simulink model "modelsimulator"  (R2023b)
settings: Solver=VariableStepAuto  StartTime=0.0  StopTime=185  FixedStep=0.0002  RelTol=1e-3
values from neighbouring files (symbols this model uses):
  eta_init = [0 0 0 0 0 0]    [Linearization_validation.m]    (also in ROV_simulation_init.m = [radius 0 0 0 0 -pi/2])
  K_full = lqr(linsysROV_lqr,Q,R)    [ROV_simulation_init.m]
  K_reduced = lqr(linsysROV_lqr_reduced_disc,Q,R)    [ROV_simulation_init.m]
  omega = 0.0174532925*5    (= 0.0872664625)    [ROV_simulation_init.m]
  p = [-125.691529893755	-8.50647884753240	275.922008410927	13.4112646958028	-226.567986780204	-3.28875901062827	118.657519470084	6.62648580653865	14.9826070833980	0.00]    [ROV_simulation_init.m]
  PID_phi = [11.6676, 5.8503, -12.3688, 0.025226,34]    [ROV_simulation_init.m]
  PID_psi = [11.3054, 1.000, -3.8005, 0.087502,30]    [ROV_simulation_init.m]
  PID_theta = [10.2974, 5.9702, -15.653, 0.016423,19]    [ROV_simulation_init.m]
  PID_x = [500.411, 30.5093, -500.8638, 0.032394,110]    [ROV_simulation_init.m]
  PID_y = [500.7275, 20.1075, -500.8002, 0.019369,110]    [ROV_simulation_init.m]
  PID_z = [500.7655, 25.0859, -500.5557, 0.026709,158]    [ROV_simulation_init.m]
  radius = 5    [ROV_simulation_init.m]
  ROV = initializeModelMatrices(m,I,COG,l,w,h,Thrusters)    [CreateGramianROV.m]    (also in CreateROVLin.m = initializeModelMatrices(m, I, COB, dim, BlueROVHeavy); Eigenvalue_tracking.m = initializeModelMatrices(m, I, COB,dim,0); Linearization_validation.m = initializeModelMatrices(m, I, COB,dim,0); ROV_simulation_init.m = initializeModelMatrices(m, Inertia, COB, dim, BlueROVHeavy))
  T_inv = ROV.T'/(ROV.T*ROV.T')    [ROV_simulation_init.m]
  ThrusterVoltage = 14    [ROV_simulation_init.m]
  v_init = [3 0 0 0 0 0]    [Linearization_validation.m]    (also in ROV_simulation_init.m = [omega omega z_rate 0 0 omega])
  z_rate = 0.1    [ROV_simulation_init.m]
libraries: simulink x60
(part 1 of 3)
settings Model: Creator=Tomas  LastModifiedBy=Ottol

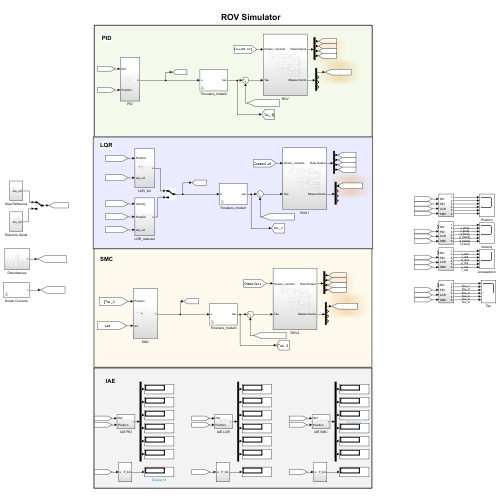
[thumbnail: Simulink's stored preview of the top-level diagram]
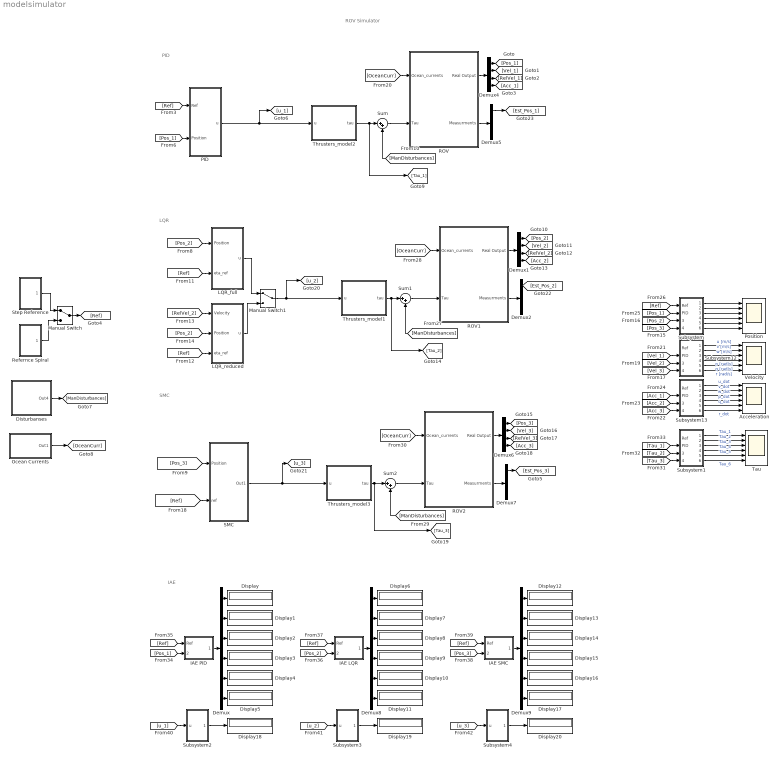
== system modelsimulator ==
  note: PID
  note: LQR
  note: SMC
  note: IAE
  note: ROV Simulator
  Acceleration : Scope  NumInputPorts=6
  Demux : Demux  Outputs=6
  Demux{1..2,4..7} (6 alike) : Demux
  Demux8 : Demux  Outputs=6
  Demux9 : Demux  Outputs=6
  Display{,1..20} (21 alike) : Display
  Disturbanses : Subsystem
  IAE LQR : Subsystem
  IAE PID : Subsystem
  IAE SMC : Subsystem
  LQR_full : Subsystem
  LQR_reduced : Subsystem
  Manual Switch : ManualSwitch
  Manual Switch1 : ManualSwitch
  Ocean Currents : Subsystem  mask{N=0, E=0, D=0}
      mask prompts: N "Current North"; E "Current East"; D "Current Down"
  PID : Subsystem
  Position : Scope  NumInputPorts=6
  ROV : Subsystem
  ROV1 : Subsystem
  ROV2 : Subsystem
  Refernce Spiral : Subsystem
  SMC : Subsystem
  Step Reference : Subsystem
  Subsystem : Subsystem
  Subsystem1 : Subsystem
  Subsystem12 : Subsystem
  Subsystem13 : Subsystem
  Subsystem2 : Subsystem
  Subsystem3 : Subsystem
  Subsystem4 : Subsystem
  Sum : Sum  Inputs=|++
  Sum1 : Sum  Inputs=|++
  Sum2 : Sum  Inputs=|++
  Tau : Scope  NumInputPorts=6
  Thrusters_model1 : Subsystem  mask{Thruster_voltage=14 V, Enable_dynamics=on}
      mask prompts: Enable_dynamics "Enable Thruster Dynamics"
      mask DialogControl DescGroupVar Prompt: T200 Thruster
      mask DialogControl DescTextVar Prompt: Thruster dynamics available for 10 to 20 V
      mask DialogControl Container3 Prompt: Thruster Voltage selection
  Thrusters_model2 : Subsystem  mask{Thruster_voltage=14 V, Enable_dynamics=on}
      mask prompts: Enable_dynamics "Enable Thruster Dynamics"
      mask DialogControl DescGroupVar Prompt: T200 Thruster
      mask DialogControl DescTextVar Prompt: Thruster dynamics available for 10 to 20 V
      mask DialogControl Container3 Prompt: Thruster Voltage selection
  Thrusters_model3 : Subsystem  mask{Thruster_voltage=14 V, Enable_dynamics=on}
      mask prompts: Enable_dynamics "Enable Thruster Dynamics"
      mask DialogControl DescGroupVar Prompt: T200 Thruster
      mask DialogControl DescTextVar Prompt: Thruster dynamics available for 10 to 20 V
      mask DialogControl Container3 Prompt: Thruster Voltage selection
  Velocity : Scope  NumInputPorts=6
  wires:
  Subsystem12/6(Out6) -> Velocity/6  "r [rad/s]"
  Subsystem12/5(Out5) -> Velocity/5  "q [rad/s]"
  Subsystem12/4(Out4) -> Velocity/4  "p [rad/s]"
  Subsystem12/3(Out3) -> Velocity/3  "w [m/s]"
  Subsystem12/2(Out2) -> Velocity/2  "v [m/s]"
  Subsystem12/1(Out1) -> Velocity/1  "u [m/s]"
  Subsystem13/1(Out1) -> Acceleration/1  "u_dot"
  Subsystem13/2(Out2) -> Acceleration/2  "v_dot"
  Subsystem13/3(Out3) -> Acceleration/3  "w_dot"
  Subsystem13/4(Out4) -> Acceleration/4  "p_dot"
  Subsystem13/5(Out5) -> Acceleration/5  "q_dot"
  Subsystem13/6(Out6) -> Acceleration/6  "r_dot"
  Sum/1 -> ROV/2(Tau)
  Thrusters_model2/1(tau) -> Sum/1, [Tau_1]
  ROV/2(Measurments) -> Demux5/1
  Subsystem/1(Out1) -> Position/1
  Subsystem/6(Out6) -> Position/6
  Subsystem/5(Out5) -> Position/5
  Subsystem/4(Out4) -> Position/4
  Subsystem/3(Out3) -> Position/3
  Subsystem/2(Out2) -> Position/2
  [Pos_1] -> PID/2(Position)
  Refernce Spiral/1(eta_ref) -> Manual Switch/2
  [Ref] -> LQR_full/2(eta_ref)
  [Ref] -> SMC/2(ref)
  Ocean Currents/1(Out1) -> [OceanCurr]
  [OceanCurr] -> ROV/1(Ocean_currents)
  Demux4/1 -> [Pos_1]
  Demux4/3 -> [RelVel_1]
  Demux4/2 -> [Vel_1]
  Demux4/4 -> [Acc_1]
  ROV/1(Real Output) -> Demux4/1
  Disturbanses/1(Out4) -> [ManDisturbances]
  [ManDisturbances] -> Sum/2
  [Pos_1] -> Subsystem/2(PID)
  [Ref] -> Subsystem/1(Ref)
  [ManDisturbances] -> Sum1/2
  ROV1/1(Real Output) -> Demux1/1
  Demux1/4 -> [Acc_2]
  Demux1/2 -> [Vel_2]
  Demux1/3 -> [RelVel_2]
  Demux1/1 -> [Pos_2]
  [OceanCurr] -> ROV1/1(Ocean_currents)
  ROV1/2(Measurments) -> Demux2/1
  Thrusters_model1/1(tau) -> [Tau_2], Sum1/1
  Sum1/1 -> ROV1/2(Tau)
  Sum2/1 -> ROV2/2(Tau)
  Thrusters_model3/1(tau) -> [Tau_3], Sum2/1
  ROV2/2(Measurments) -> Demux7/1
  [OceanCurr] -> ROV2/1(Ocean_currents)
  Demux6/1 -> [Pos_3]
  Demux6/3 -> [RelVel_3]
  Demux6/2 -> [Vel_3]
  Demux6/4 -> [Acc_3]
  ROV2/1(Real Output) -> Demux6/1
  [ManDisturbances] -> Sum2/2
  Step Reference/1(eta_ref) -> Manual Switch/1
  Manual Switch/1 -> [Ref]
  [Ref] -> PID/1(Ref)
  [Pos_2] -> LQR_full/1(Position)
  [Pos_3] -> SMC/1(Position)
  [Pos_2] -> LQR_reduced/2(Position)
  [RelVel_2] -> LQR_reduced/1(Velocity)
  [Ref] -> LQR_reduced/3(eta_ref)
  LQR_full/1(u) -> Manual Switch1/1
  LQR_reduced/1(u) -> Manual Switch1/2
  [Pos_3] -> Subsystem/4(SMC)
  [Vel_1] -> Subsystem12/2(PID)
  [Vel_2] -> Subsystem12/3(LQR)
  [Vel_3] -> Subsystem12/4(SMC)
  [Acc_1] -> Subsystem13/2(PID)
  [Acc_2] -> Subsystem13/3(LQR)
  [Acc_3] -> Subsystem13/4(SMC)
  [Tau_2] -> Subsystem1/3(LQR)
  Subsystem1/5(Out5) -> Tau/5  "Tau_5"
  Subsystem1/6(Out6) -> Tau/6  "Tau_6"
  Subsystem1/4(Out4) -> Tau/4  "Tau_4"
  Subsystem1/3(Out3) -> Tau/3  "Tau_3"
  [Tau_1] -> Subsystem1/2(PID)
  Subsystem1/1(Out1) -> Tau/1  "Tau_1"
  [Tau_3] -> Subsystem1/4(SMC)
  Subsystem1/2(Out2) -> Tau/2  "Tau_2"
  Demux/3 -> Display2/1
  Demux/1 -> Display/1
  Demux/6 -> Display5/1
  Demux/4 -> Display3/1
  Demux/2 -> Display1/1
  Demux/5 -> Display4/1
  IAE PID/1(Out1) -> Demux/1
  [Ref] -> IAE PID/1(Ref)
  [Pos_1] -> IAE PID/2(Position)
  Demux8/5 -> Display10/1
  Demux8/2 -> Display7/1
  Demux8/3 -> Display8/1
  Demux8/1 -> Display6/1
  IAE LQR/1(Out1) -> Demux8/1
  Demux8/6 -> Display11/1
  [Pos_2] -> IAE LQR/2(Position)
  Demux8/4 -> Display9/1
  [Ref] -> IAE LQR/1(Ref)
  Demux9/5 -> Display16/1
  Demux9/2 -> Display13/1
  Demux9/3 -> Display14/1
  Demux9/1 -> Display12/1
  IAE SMC/1(Out1) -> Demux9/1
  Demux9/6 -> Display17/1
  [Pos_3] -> IAE SMC/2(Position)
  Demux9/4 -> Display15/1
  [Ref] -> IAE SMC/1(Ref)
  [Pos_2] -> Subsystem/3(LQR)
  SMC/1(Out1) -> [u_3], Thrusters_model3/1(u)
  Manual Switch1/1 -> [u_2], Thrusters_model1/1(u)
  PID/1(u) -> Thrusters_model2/1(u), [u_1]
  [u_1] -> Subsystem2/1(u)
  Subsystem2/1(F_tot) -> Display18/1
  [u_2] -> Subsystem3/1(u)
  Subsystem3/1(F_tot) -> Display19/1
  [u_3] -> Subsystem4/1(u)
  Subsystem4/1(F_tot) -> Display20/1
  Demux7/1 -> [Est_Pos_3]
  Demux2/1 -> [Est_Pos_2]
  Demux5/1 -> [Est_Pos_1]

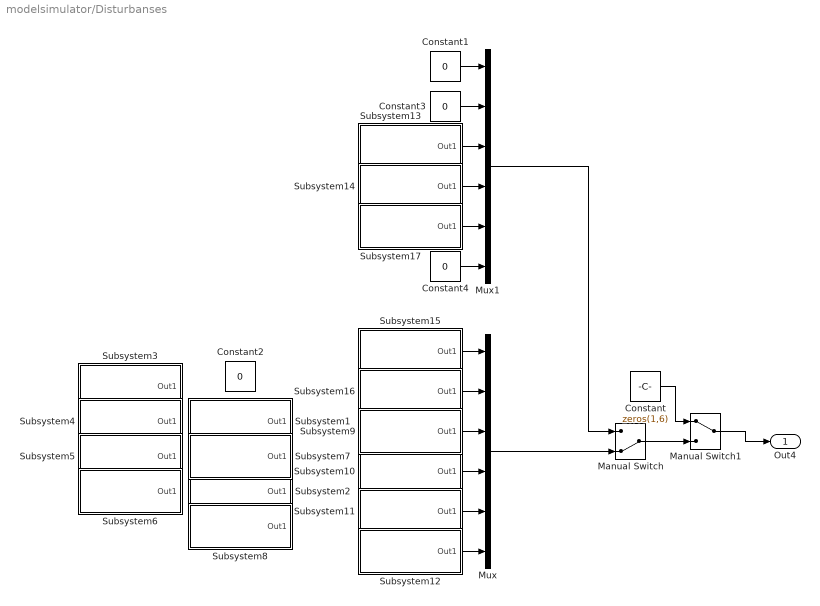
== system modelsimulator/Disturbanses ==
  Constant : Constant  Value=zeros(1,6)
  Constant{1..4} (4 alike) : Constant  Value=0
  Manual Switch : ManualSwitch  CurrentSetting=0
  Manual Switch1 : ManualSwitch
  Mux : Mux  Inputs=6
  Mux1 : Mux  Inputs=6
  Subsystem1 : Subsystem  mask{Step_time_1=5, Step_time_2=20, Init_val=0, New_val=100}
      mask prompts: Step_time_1 "Step time 1:"; Step_time_2 "Step time 2:"; Init_val "Inital Value:"; New_val "New Value:"
      mask Display: plot([1 2 3 4 4 5 6 7 7 8 9 10],[0 0 0 0 1 1 1 1 0 0 0 0]);
  Subsystem10 : Subsystem  mask{Step_time_1=95, Step_time_2=110, Init_val=0, New_val=1}
      mask prompts: Step_time_1 "Step time 1:"; Step_time_2 "Step time 2:"; Init_val "Inital Value:"; New_val "New Value:"
      mask Display: plot([1 2 3 4 4 5 6 7 7 8 9 10],[0 0 0 0 1 1 1 1 0 0 0 0]);
  Subsystem11 : Subsystem  mask{Step_time_1=125, Step_time_2=140, Init_val=0, New_val=1}
      mask prompts: Step_time_1 "Step time 1:"; Step_time_2 "Step time 2:"; Init_val "Inital Value:"; New_val "New Value:"
      mask Display: plot([1 2 3 4 4 5 6 7 7 8 9 10],[0 0 0 0 1 1 1 1 0 0 0 0]);
  Subsystem12 : Subsystem  mask{Step_time_1=155, Step_time_2=170, Init_val=0, New_val=1}
      mask prompts: Step_time_1 "Step time 1:"; Step_time_2 "Step time 2:"; Init_val "Inital Value:"; New_val "New Value:"
      mask Display: plot([1 2 3 4 4 5 6 7 7 8 9 10],[0 0 0 0 1 1 1 1 0 0 0 0]);
  Subsystem13 : Subsystem  mask{Step_time_1=95, Step_time_2=110, Init_val=0, New_val=10}
      mask prompts: Step_time_1 "Step time 1:"; Step_time_2 "Step time 2:"; Init_val "Inital Value:"; New_val "New Value:"
      mask Display: plot([1 2 3 4 4 5 6 7 7 8 9 10],[0 0 0 0 1 1 1 1 0 0 0 0]);
  Subsystem14 : Subsystem  mask{Step_time_1=125, Step_time_2=140, Init_val=0, New_val=1}
      mask prompts: Step_time_1 "Step time 1:"; Step_time_2 "Step time 2:"; Init_val "Inital Value:"; New_val "New Value:"
      mask Display: plot([1 2 3 4 4 5 6 7 7 8 9 10],[0 0 0 0 1 1 1 1 0 0 0 0]);
  Subsystem15 : Subsystem  mask{Step_time_1=5, Step_time_2=20, Init_val=0, New_val=10}
      mask prompts: Step_time_1 "Step time 1:"; Step_time_2 "Step time 2:"; Init_val "Inital Value:"; New_val "New Value:"
      mask Display: plot([1 2 3 4 4 5 6 7 7 8 9 10],[0 0 0 0 1 1 1 1 0 0 0 0]);
  Subsystem16 : Subsystem  mask{Step_time_1=35, Step_time_2=50, Init_val=0, New_val=10}
      mask prompts: Step_time_1 "Step time 1:"; Step_time_2 "Step time 2:"; Init_val "Inital Value:"; New_val "New Value:"
      mask Display: plot([1 2 3 4 4 5 6 7 7 8 9 10],[0 0 0 0 1 1 1 1 0 0 0 0]);
  Subsystem17 : Subsystem  mask{Step_time_1=155, Step_time_2=170, Init_val=0, New_val=1}
      mask prompts: Step_time_1 "Step time 1:"; Step_time_2 "Step time 2:"; Init_val "Inital Value:"; New_val "New Value:"
      mask Display: plot([1 2 3 4 4 5 6 7 7 8 9 10],[0 0 0 0 1 1 1 1 0 0 0 0]);
  Subsystem2 : Subsystem  mask{Step_time_1=65, Step_time_2=80, Init_val=0, New_val=1}
      mask prompts: Step_time_1 "Step time 1:"; Step_time_2 "Step time 2:"; Init_val "Inital Value:"; New_val "New Value:"
      mask Display: plot([1 2 3 4 4 5 6 7 7 8 9 10],[0 0 0 0 1 1 1 1 0 0 0 0]);
  Subsystem3 : Subsystem  mask{Step_time_1=14, Step_time_2=16, Init_val=0, New_val=5}
      mask prompts: Step_time_1 "Step time 1:"; Step_time_2 "Step time 2:"; Init_val "Inital Value:"; New_val "New Value:"
      mask Display: plot([1 2 3 4 4 5 6 7 7 8 9 10],[0 0 0 0 1 1 1 1 0 0 0 0]);
  Subsystem4 : Subsystem  mask{Step_time_1=20, Step_time_2=22, Init_val=0, New_val=1}
      mask prompts: Step_time_1 "Step time 1:"; Step_time_2 "Step time 2:"; Init_val "Inital Value:"; New_val "New Value:"
      mask Display: plot([1 2 3 4 4 5 6 7 7 8 9 10],[0 0 0 0 1 1 1 1 0 0 0 0]);
  Subsystem5 : Subsystem  mask{Step_time_1=26, Step_time_2=28, Init_val=0, New_val=1}
      mask prompts: Step_time_1 "Step time 1:"; Step_time_2 "Step time 2:"; Init_val "Inital Value:"; New_val "New Value:"
      mask Display: plot([1 2 3 4 4 5 6 7 7 8 9 10],[0 0 0 0 1 1 1 1 0 0 0 0]);
  Subsystem6 : Subsystem  mask{Step_time_1=32, Step_time_2=34, Init_val=0, New_val=1}
      mask prompts: Step_time_1 "Step time 1:"; Step_time_2 "Step time 2:"; Init_val "Inital Value:"; New_val "New Value:"
      mask Display: plot([1 2 3 4 4 5 6 7 7 8 9 10],[0 0 0 0 1 1 1 1 0 0 0 0]);
  Subsystem7 : Subsystem  mask{Step_time_1=35, Step_time_2=50, Init_val=0, New_val=10}
      mask prompts: Step_time_1 "Step time 1:"; Step_time_2 "Step time 2:"; Init_val "Inital Value:"; New_val "New Value:"
      mask Display: plot([1 2 3 4 4 5 6 7 7 8 9 10],[0 0 0 0 1 1 1 1 0 0 0 0]);
  Subsystem8 : Subsystem  mask{Step_time_1=95, Step_time_2=110, Init_val=0, New_val=10}
      mask prompts: Step_time_1 "Step time 1:"; Step_time_2 "Step time 2:"; Init_val "Inital Value:"; New_val "New Value:"
      mask Display: plot([1 2 3 4 4 5 6 7 7 8 9 10],[0 0 0 0 1 1 1 1 0 0 0 0]);
  Subsystem9 : Subsystem  mask{Step_time_1=65, Step_time_2=80, Init_val=0, New_val=10}
      mask prompts: Step_time_1 "Step time 1:"; Step_time_2 "Step time 2:"; Init_val "Inital Value:"; New_val "New Value:"
      mask Display: plot([1 2 3 4 4 5 6 7 7 8 9 10],[0 0 0 0 1 1 1 1 0 0 0 0]);
  Out4 : Outport
  wires:
  Subsystem9/1(Out1) -> Mux/3
  Subsystem15/1(Out1) -> Mux/1
  Subsystem16/1(Out1) -> Mux/2
  Subsystem10/1(Out1) -> Mux/4
  Subsystem11/1(Out1) -> Mux/5
  Subsystem12/1(Out1) -> Mux/6
  Subsystem13/1(Out1) -> Mux1/3
  Subsystem14/1(Out1) -> Mux1/4
  Subsystem17/1(Out1) -> Mux1/5
  Constant1/1 -> Mux1/1
  Constant3/1 -> Mux1/2
  Constant4/1 -> Mux1/6
  Mux/1 -> Manual Switch/2
  Mux1/1 -> Manual Switch/1
  Manual Switch/1 -> Manual Switch1/2
  Manual Switch1/1 -> Out4/1
  Constant/1 -> Manual Switch1/1

== system modelsimulator/IAE LQR ==
  Ref : Inport
  Position : Inport  Port=2
  Abs : Abs  SaturateOnIntegerOverflow=off
  Integrator : Integrator
  Sum : Sum  Inputs=|+-
  Out1 : Outport
  wires:
  Ref/1 -> Sum/1
  Position/1 -> Sum/2
  Sum/1 -> Abs/1
  Abs/1 -> Integrator/1
  Integrator/1 -> Out1/1

== system modelsimulator/IAE PID ==
  Ref : Inport
  Position : Inport  Port=2
  Abs : Abs  SaturateOnIntegerOverflow=off
  Integrator : Integrator
  Sum : Sum  Inputs=|+-
  Out1 : Outport
  wires:
  Ref/1 -> Sum/1
  Position/1 -> Sum/2
  Sum/1 -> Abs/1
  Abs/1 -> Integrator/1
  Integrator/1 -> Out1/1

== system modelsimulator/IAE SMC ==
  Ref : Inport
  Position : Inport  Port=2
  Abs : Abs  SaturateOnIntegerOverflow=off
  Integrator : Integrator
  Sum : Sum  Inputs=|+-
  Out1 : Outport
  wires:
  Ref/1 -> Sum/1
  Position/1 -> Sum/2
  Sum/1 -> Abs/1
  Abs/1 -> Integrator/1
  Integrator/1 -> Out1/1

== system modelsimulator/LQR_full ==
  Position : Inport  PortDimensions=6
  eta_ref : Inport  Port=2  PortDimensions=6
  Constant7 : Constant  Value=-K_full
  Demux : Demux  Outputs=6
  Demux1 : Demux  Outputs=6
  Demux2 : Demux  Outputs=6
  Discrete Derivative2 : simulink/Discrete/Discrete Derivative  gainval=1.0  ICPrevScaledInput=0.0  OutMin=[]  OutMax=[]  OutDataType=fixdt(1, 16)  OutScaling=2^-10  DoSatur=off
  Force allocation : Subsystem  mask{Thruster_voltage=14 V, upper_sat=44, lower_sat=34, Enable_dynamics=on}
      mask prompts: upper_sat "Upper saturation"; lower_sat "Lower saturation"; Enable_dynamics "Enable Thruster Dynamics"
      mask DialogControl DescGroupVar Prompt: T200 Thruster
      mask DialogControl DescTextVar Prompt: Thruster dynamics available for 10 to 20 V
      mask DialogControl Container3 Prompt: Thruster Voltage selection
  Integrator : Integrator
  Matrix Multiply : Product  Multiplication=Matrix(*)
  Mux : Mux  Inputs=18
  Saturation : Saturate  UpperLimit=1  LowerLimit=-1
  Subsystem : Subsystem
  Sum : Sum  Inputs=+-|
  Sum1 : Sum  Inputs=|++
  Tau_body : Subsystem
  Zero-Order Hold1 : ZeroOrderHold  SampleTime=1/20
  Zero-Order Hold2 : ZeroOrderHold  SampleTime=1/20
  Zero-Order Hold4 : ZeroOrderHold  SampleTime=1/20
  u : Outport
  wires:
  Force allocation/1(u) -> Zero-Order Hold4/1
  Constant7/1 -> Matrix Multiply/1
  Sum/1 -> Integrator/1, Demux1/1
  eta_ref/1 -> Zero-Order Hold2/1
  Demux/1 -> Mux/1
  Demux/2 -> Mux/2
  Demux/3 -> Mux/3
  Demux/4 -> Mux/4
  Demux/5 -> Mux/5
  Demux/6 -> Mux/6
  Demux1/1 -> Mux/7
  Demux1/2 -> Mux/8
  Demux1/3 -> Mux/9
  Demux1/4 -> Mux/10
  Demux1/5 -> Mux/11
  Demux1/6 -> Mux/12
  Demux2/1 -> Mux/13
  Demux2/2 -> Mux/14
  Demux2/3 -> Mux/15
  Demux2/4 -> Mux/16
  Demux2/5 -> Mux/17
  Demux2/6 -> Mux/18
  Integrator/1 -> Demux2/1
  Position/1 -> Tau_body/2(Pos), Zero-Order Hold1/1
  Mux/1 -> Matrix Multiply/2
  Zero-Order Hold2/1 -> Subsystem/1(eta_ref), Sum/2
  Zero-Order Hold1/1 -> Sum/1, Discrete Derivative2/1
  Zero-Order Hold4/1 -> Saturation/1
  Saturation/1 -> u/1
  Tau_body/1(Tau_b) -> Force allocation/1(Tau)
  Matrix Multiply/1 -> Sum1/1
  Sum1/1 -> Tau_body/1(Tau)
  Subsystem/1(Out1) -> Sum1/2
  Discrete Derivative2/1 -> Demux/1

== system modelsimulator/LQR_reduced ==
  Velocity : Inport  PortDimensions=6
  Position : Inport  Port=2  PortDimensions=6
  eta_ref : Inport  Port=3  PortDimensions=6
  Constant7 : Constant  Value=-K_reduced
  Demux1 : Demux  Outputs=6
  Demux2 : Demux  Outputs=6
  Demux3 : Demux  Outputs=6
  Force allocation : Subsystem  mask{Thruster_voltage=14 V, upper_sat=44, lower_sat=34, Enable_dynamics=on}
      mask prompts: upper_sat "Upper saturation"; lower_sat "Lower saturation"; Enable_dynamics "Enable Thruster Dynamics"
      mask DialogControl DescGroupVar Prompt: T200 Thruster
      mask DialogControl DescTextVar Prompt: Thruster dynamics available for 10 to 20 V
      mask DialogControl Container3 Prompt: Thruster Voltage selection
  Integrator : Integrator
  Matrix Multiply : Product  Multiplication=Matrix(*)
  Mux : Mux  Inputs=9
  Saturation : Saturate  UpperLimit=1  LowerLimit=-1
  Subsystem : Subsystem
  Sum : Sum  Inputs=+-|
  Sum1 : Sum  Inputs=|++
  Zero-Order Hold{,1..3} (4 alike) : ZeroOrderHold  SampleTime=1/20
  u : Outport
  wires:
  Force allocation/1(u) -> Zero-Order Hold/1
  Constant7/1 -> Matrix Multiply/1
  Sum/1 -> Demux1/1, Integrator/1
  eta_ref/1 -> Subsystem/1(eta_ref), Zero-Order Hold3/1
  Integrator/1 -> Demux2/1
  Position/1 -> Zero-Order Hold2/1
  Mux/1 -> Matrix Multiply/2
  Velocity/1 -> Zero-Order Hold1/1
  Demux3/3 -> Mux/1
  Demux3/4 -> Mux/2
  Demux3/5 -> Mux/3
  Demux1/3 -> Mux/4
  Demux1/4 -> Mux/5
  Demux1/5 -> Mux/6
  Demux2/3 -> Mux/7
  Demux2/4 -> Mux/8
  Demux2/5 -> Mux/9
  Zero-Order Hold/1 -> Saturation/1
  Zero-Order Hold1/1 -> Demux3/1
  Zero-Order Hold2/1 -> Sum/1
  Zero-Order Hold3/1 -> Sum/2
  Saturation/1 -> u/1
  Sum1/1 -> Force allocation/1(Tau)
  Matrix Multiply/1 -> Sum1/1
  Subsystem/1(Out1) -> Sum1/2

== system modelsimulator/Ocean Currents ==
  Constant : Constant  Value=0
  Constant1 : Constant  Value=D
  Constant2 : Constant  Value=E
  Constant3 : Constant  Value=N
  Mux : Mux  Inputs=6
  Out1 : Outport
  wires:
  Constant3/1 -> Mux/1
  Constant/1 -> Mux/6, Mux/4, Mux/5
  Mux/1 -> Out1/1
  Constant2/1 -> Mux/2
  Constant1/1 -> Mux/3

== system modelsimulator/PID ==
  Ref : Inport
  Position : Inport  Port=2
  Constant : Constant  Value=0
  Constant1 : Constant  Value=0
  Constant2 : Constant  Value=0
  Demux1 : Demux  Outputs=6
  Demux4 : Demux  Outputs=6
  Force allocation : Subsystem  mask{Thruster_voltage=14 V, upper_sat=44, lower_sat=34, Enable_dynamics=on}
      mask prompts: upper_sat "Upper saturation"; lower_sat "Lower saturation"; Enable_dynamics "Enable Thruster Dynamics"
      mask DialogControl DescGroupVar Prompt: T200 Thruster
      mask DialogControl DescTextVar Prompt: Thruster dynamics available for 10 to 20 V
      mask DialogControl Container3 Prompt: Thruster Voltage selection
  G1 : Subsystem  mask{Kc=PID_x(1), Ki=PID_x(2), Kd=PID_x(3), Tf=PID_x(4), umax=PID_x(5), Arb_pnk=0, Init=0}
      mask prompts: umax "Max/Min u"; Arb_pnk "Arbeidspunkt"; Init "Initialverdi"
  G2 : Subsystem  mask{Kc=PID_y(1), Ki=PID_y(2), Kd=PID_y(3), Tf=PID_y(4), umax=PID_y(5), Arb_pnk=0, Init=0}
      mask prompts: umax "Max/Min u"; Arb_pnk "Arbeidspunkt"; Init "Initialverdi"
  G3 : Subsystem  mask{Kc=PID_z(1), Ki=PID_z(2), Kd=PID_z(3), Tf=PID_z(4), umax=PID_z(5), Arb_pnk=0, Init=0}
      mask prompts: umax "Max/Min u"; Arb_pnk "Arbeidspunkt"; Init "Initialverdi"
  G4 : Subsystem  mask{Kc=PID_phi(1), Ki=PID_phi(2), Kd=PID_phi(3), Tf=PID_phi(4), umax=PID_phi(5), Arb_pnk=0, Init=0}
      mask prompts: umax "Max/Min u"; Arb_pnk "Arbeidspunkt"; Init "Initialverdi"
  G5 : Subsystem  mask{Kc=PID_theta(1), Ki=PID_theta(2), Kd=PID_theta(3), Tf=PID_theta(4), umax=PID_theta(5), Arb_pnk=0, Init=0}
      mask prompts: umax "Max/Min u"; Arb_pnk "Arbeidspunkt"; Init "Initialverdi"
  G6 : Subsystem  mask{Kc=PID_psi(1), Ki=PID_psi(2), Kd=PID_psi(3), Tf=PID_psi(4), umax=PID_psi(5), Arb_pnk=0, Init=0}
      mask prompts: umax "Max/Min u"; Arb_pnk "Arbeidspunkt"; Init "Initialverdi"
  Manual Switch : ManualSwitch  CurrentSetting=0
  Manual Switch1 : ManualSwitch  CurrentSetting=0
  Manual Switch2 : ManualSwitch  CurrentSetting=0
  Mux : Mux  Inputs=6
  Saturation : Saturate  UpperLimit=1  LowerLimit=-1
  Tau_body : Subsystem
  Zero-Order Hold : ZeroOrderHold  SampleTime=1/20
  Zero-Order Hold1 : ZeroOrderHold  SampleTime=1/20
  Zero-Order Hold2 : ZeroOrderHold  SampleTime=1/20
  u : Outport
  wires:
  Demux4/4 -> G4/1(ref)  "Phi [rad]"
  Position/1 -> Zero-Order Hold1/1
  Demux4/6 -> G6/1(ref)  "Psi [rad]"
  Demux4/5 -> G5/1(ref)  "Theta [rad]"
  Demux4/3 -> G3/1(ref)  "z [m]"
  Ref/1 -> Zero-Order Hold/1
  Force allocation/1(u) -> Zero-Order Hold2/1
  Demux4/2 -> G2/1(ref)  "y [m]"
  Demux4/1 -> G1/1(ref)  "x [m]"
  Mux/1 -> Tau_body/1(Tau)
  Tau_body/1(Tau_b) -> Force allocation/1(Tau)
  Manual Switch/1 -> Mux/1
  G1/1(u) -> Manual Switch/2
  Constant/1 -> Manual Switch/1
  Constant1/1 -> Manual Switch1/1
  G2/1(u) -> Manual Switch1/2
  Manual Switch1/1 -> Mux/2
  G3/1(u) -> Mux/3
  G4/1(u) -> Mux/4
  G5/1(u) -> Mux/5
  Zero-Order Hold1/1 -> Demux1/1, Tau_body/2(Pos)
  G6/1(u) -> Manual Switch2/2
  Constant2/1 -> Manual Switch2/1
  Manual Switch2/1 -> Mux/6
  Zero-Order Hold2/1 -> Saturation/1
  Zero-Order Hold/1 -> Demux4/1
  Demux1/1 -> G1/2(position)  "x [m]"
  Demux1/2 -> G2/2(position)  "y [m]"
  Demux1/3 -> G3/2(position)  "z [m]"
  Demux1/4 -> G4/2(position)  "Phi [rad]"
  Demux1/5 -> G5/2(position)  "Theta [rad]"
  Demux1/6 -> G6/2(position)  "Psi [rad]"
  Saturation/1 -> u/1

== system modelsimulator/ROV ==
  Ocean_currents : Inport
  Tau : Inport  Port=2
  Integrator : Integrator  InitialCondition=v_init
  Integrator1 : Integrator  InitialCondition=eta_init
  Integrator2 : Integrator  InitialCondition=v_init
  Integrator3 : Integrator  InitialCondition=eta_init
  Measurement Noise : Subsystem
  Measurement Noise1 : Subsystem
  Measurement Noise2 : Subsystem
  Mux : Mux
  Mux1 : Mux
  NED : Subsystem
  NED1 : Subsystem
  ROVSubsystem : Subsystem
  Sum : Sum  Inputs=++|
  Sum1 : Sum  Inputs=++|
  Real Output : Outport
  Measurments : Outport  Port=2
  wires:
  Integrator1/1 -> NED/2(position_NED), Mux/1, ROVSubsystem/2(Position)  "Position"
  ROVSubsystem/1(Acceleration) -> Mux/4, Integrator/1, Measurement Noise/1(In1)  "Acceleration"
  Tau/1 -> ROVSubsystem/3(Tau)
  NED/1(Velocity_NED) -> Integrator1/1  "ned_d"
  Sum/1 -> Mux/2, NED/1(velocity)  "Velocity"
  Integrator/1 -> Mux/3, Sum/2, ROVSubsystem/1(Velocity)  "RelVelo"
  Measurement Noise1/1(EstVelo) -> Mux1/3, Sum1/2  "EstRelVelo"
  Sum1/1 -> Mux1/2, NED1/1(velocity)  "EstVelo"
  NED1/1(Velocity_NED) -> Integrator3/1
  Measurement Noise2/1(EstPos) -> NED1/2(position_NED), Mux1/1  "EstPos"
  Measurement Noise/1(EstAcc) -> Integrator2/1, Mux1/4  "EstAcc"
  [OceanCurrent] -> Sum1/1
  [OceanCurrent] -> Sum/1
  Ocean_currents/1 -> [OceanCurrent]
  Mux/1 -> Real Output/1
  Mux1/1 -> Measurments/1
  Integrator2/1 -> Measurement Noise1/1(In1)
  Integrator3/1 -> Measurement Noise2/1(In1)

== system modelsimulator/ROV1 ==
  Ocean_currents : Inport
  Tau : Inport  Port=2
  Integrator : Integrator  InitialCondition=v_init
  Integrator1 : Integrator  InitialCondition=eta_init
  Integrator2 : Integrator  InitialCondition=v_init
  Integrator3 : Integrator  InitialCondition=eta_init
  Measurement Noise : Subsystem
  Measurement Noise1 : Subsystem
  Measurement Noise2 : Subsystem
  Mux : Mux
  Mux1 : Mux
  NED : Subsystem
  NED1 : Subsystem
  ROVSubsystem : Subsystem
  Sum : Sum  Inputs=++|
  Sum1 : Sum  Inputs=++|
  Real Output : Outport
  Measurments : Outport  Port=2
  wires:
  Integrator3/1 -> Measurement Noise2/1(In1)
  Integrator2/1 -> Measurement Noise1/1(In1)
  Mux1/1 -> Measurments/1
  Mux/1 -> Real Output/1
  Ocean_currents/1 -> [OceanCurrent]
  [OceanCurrent] -> Sum/1
  [OceanCurrent] -> Sum1/1
  Measurement Noise/1(EstAcc) -> Mux1/4, Integrator2/1  "EstAcc"
  Measurement Noise2/1(EstPos) -> Mux1/1, NED1/2(position_NED)  "EstPos"
  NED1/1(Velocity_NED) -> Integrator3/1
  Sum1/1 -> NED1/1(velocity), Mux1/2  "EstVelo"
  Measurement Noise1/1(EstVelo) -> Sum1/2, Mux1/3  "EstRelVelo"
  Integrator/1 -> ROVSubsystem/1(Velocity), Sum/2, Mux/3  "RelVelo"
  Sum/1 -> NED/1(velocity), Mux/2  "Velocity"
  NED/1(Velocity_NED) -> Integrator1/1  "ned_d"
  Tau/1 -> ROVSubsystem/3(Tau)
  ROVSubsystem/1(Acceleration) -> Measurement Noise/1(In1), Integrator/1, Mux/4  "Acceleration"
  Integrator1/1 -> ROVSubsystem/2(Position), Mux/1, NED/2(position_NED)  "Position"

== system modelsimulator/ROV2 ==
  Ocean_currents : Inport
  Tau : Inport  Port=2
  Integrator : Integrator  InitialCondition=v_init
  Integrator1 : Integrator  InitialCondition=eta_init
  Integrator2 : Integrator  InitialCondition=v_init
  Integrator3 : Integrator  InitialCondition=eta_init
  Measurement Noise : Subsystem
  Measurement Noise1 : Subsystem
  Measurement Noise2 : Subsystem
  Mux : Mux
  Mux1 : Mux
  NED : Subsystem
  NED1 : Subsystem
  ROVSubsystem : Subsystem
  Sum : Sum  Inputs=++|
  Sum1 : Sum  Inputs=++|
  Real Output : Outport
  Measurments : Outport  Port=2
  wires:
  Integrator1/1 -> NED/2(position_NED), Mux/1, ROVSubsystem/2(Position)  "Position"
  ROVSubsystem/1(Acceleration) -> Mux/4, Integrator/1, Measurement Noise/1(In1)  "Acceleration"
  Tau/1 -> ROVSubsystem/3(Tau)
  NED/1(Velocity_NED) -> Integrator1/1  "ned_d"
  Sum/1 -> Mux/2, NED/1(velocity)  "Velocity"
  Integrator/1 -> Mux/3, Sum/2, ROVSubsystem/1(Velocity)  "RelVelo"
  Measurement Noise1/1(EstVelo) -> Mux1/3, Sum1/2  "EstRelVelo"
  Sum1/1 -> Mux1/2, NED1/1(velocity)  "EstVelo"
  NED1/1(Velocity_NED) -> Integrator3/1
  Measurement Noise2/1(EstPos) -> NED1/2(position_NED), Mux1/1  "EstPos"
  Measurement Noise/1(EstAcc) -> Integrator2/1, Mux1/4  "EstAcc"
  [OceanCurrent] -> Sum1/1
  [OceanCurrent] -> Sum/1
  Ocean_currents/1 -> [OceanCurrent]
  Mux/1 -> Real Output/1
  Mux1/1 -> Measurments/1
  Integrator2/1 -> Measurement Noise1/1(In1)
  Integrator3/1 -> Measurement Noise2/1(In1)

== system modelsimulator/Refernce Spiral ==
  Constant1 : Constant  Value=-pi/2
  Constant4 : Constant  Value=0
  Constant5 : Constant  Value=0
  Cos : Trigonometry
  Gain : Gain  Gain=radius
  Gain1 : Gain  Gain=radius
  Mux3 : Mux  Inputs=6
  Ramp : simulink/Sources/Ramp  slope=omega  start=0  InitialOutput=0
  Ramp1 : simulink/Sources/Ramp  slope=z_rate  start=0  InitialOutput=0
  Sin : Trigonometry  Operator=cos
  Sum : Sum  Inputs=|++
  eta_ref : Outport
  wires:
  Ramp/1 -> Cos/1, Sum/1, Sin/1
  Constant5/1 -> Mux3/5
  Constant4/1 -> Mux3/4
  Ramp1/1 -> Mux3/3
  Mux3/1 -> eta_ref/1
  Cos/1 -> Gain1/1
  Sin/1 -> Gain/1
  Constant1/1 -> Sum/2
  Gain/1 -> Mux3/1
  Gain1/1 -> Mux3/2
  Sum/1 -> Mux3/6

== system modelsimulator/SMC ==
  Position : Inport
  ref : Inport  Port=2
  Demux : Demux  Outputs=6
  Discrete Derivative : simulink/Discrete/Discrete Derivative  gainval=1.0  ICPrevScaledInput=0.0  OutMin=[]  OutMax=[]  OutDataType=fixdt(1, 16)  OutScaling=2^-10  DoSatur=off
  Discrete Derivative1 : simulink/Discrete/Discrete Derivative  gainval=1.0  ICPrevScaledInput=0.0  OutMin=[]  OutMax=[]  OutDataType=fixdt(1, 16)  OutScaling=2^-10  DoSatur=off
  Discrete Derivative2 : simulink/Discrete/Discrete Derivative  gainval=1.0  ICPrevScaledInput=0.0  OutMin=[]  OutMax=[]  OutDataType=fixdt(1, 16)  OutScaling=2^-10  DoSatur=off
  Force allocation : Subsystem  mask{Thruster_voltage=14 V, upper_sat=44, lower_sat=34, Enable_dynamics=on}
      mask prompts: upper_sat "Upper saturation"; lower_sat "Lower saturation"; Enable_dynamics "Enable Thruster Dynamics"
      mask DialogControl DescGroupVar Prompt: T200 Thruster
      mask DialogControl DescTextVar Prompt: Thruster dynamics available for 10 to 20 V
      mask DialogControl Container3 Prompt: Thruster Voltage selection
  Integrator : Integrator
  Mux : Mux  Inputs=6
  SMC_internal : Subsystem
  Saturation : Saturate  UpperLimit=1  LowerLimit=-1
  Sum : Sum  Inputs=|+-
  Tau_body : Subsystem
  Zero-Order Hold : ZeroOrderHold  SampleTime=1/20
  Zero-Order Hold1 : ZeroOrderHold  SampleTime=1/20
  Zero-Order Hold2 : ZeroOrderHold  SampleTime=1/20
  Out1 : Outport
  wires:
  SMC_internal/1(Tau) -> Tau_body/2(Tau)
  ref/1 -> Zero-Order Hold/1
  Discrete Derivative/1 -> SMC_internal/5(Ref_dd)
  Force allocation/1(u) -> Zero-Order Hold1/1
  Tau_body/1(Tau_b) -> Force allocation/1(Tau)
  Discrete Derivative1/1 -> Discrete Derivative/1, SMC_internal/4(Ref_d)
  Zero-Order Hold/1 -> Sum/2, Discrete Derivative1/1, SMC_internal/3(Ref)
  Discrete Derivative2/1 -> SMC_internal/2(Velocity)
  Sum/1 -> Integrator/1
  Integrator/1 -> SMC_internal/6(e_int)
  Zero-Order Hold1/1 -> Saturation/1
  Saturation/1 -> Out1/1
  Zero-Order Hold2/1 -> Tau_body/1(Pos), SMC_internal/1(Position), Discrete Derivative2/1, Sum/1
  Position/1 -> Demux/1
  Demux/3 -> Mux/3
  Demux/4 -> Mux/4
  Demux/5 -> Mux/5
  Mux/1 -> Zero-Order Hold2/1
  Demux/2 -> Mux/2
  Demux/1 -> Mux/1
  Demux/6 -> Mux/6

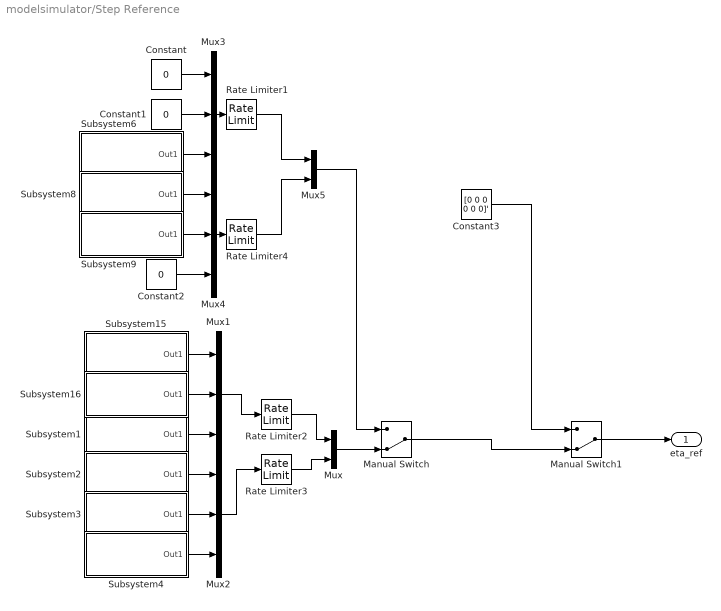
== system modelsimulator/Step Reference ==
  Constant : Constant  Value=0
  Constant1 : Constant  Value=0
  Constant2 : Constant  Value=0
  Constant3 : Constant  Value=[0 0 0 0 0 0]'
  Manual Switch : ManualSwitch  CurrentSetting=0
  Manual Switch1 : ManualSwitch  CurrentSetting=0
  Mux : Mux  Inputs=2
  Mux{1..4} (4 alike) : Mux  Inputs=3
  Mux5 : Mux  Inputs=2
  Rate Limiter1 : RateLimiter  RisingSlewLimit=0.5  FallingSlewLimit=-0.5  SampleTimeMode=inherited
  Rate Limiter2 : RateLimiter  RisingSlewLimit=0.4  FallingSlewLimit=-0.4  SampleTimeMode=inherited
  Rate Limiter3 : RateLimiter  RisingSlewLimit=0.5  FallingSlewLimit=-0.5  SampleTimeMode=inherited
  Rate Limiter4 : RateLimiter  RisingSlewLimit=0.5  FallingSlewLimit=-0.5  SampleTimeMode=inherited
  Subsystem1 : Subsystem  mask{Step_time_1=65, Step_time_2=80, Init_val=0, New_val=1}
      mask prompts: Step_time_1 "Step time 1:"; Step_time_2 "Step time 2:"; Init_val "Inital Value:"; New_val "New Value:"
      mask Display: plot([1 2 3 4 4 5 6 7 7 8 9 10],[0 0 0 0 1 1 1 1 0 0 0 0]);
  Subsystem15 : Subsystem  mask{Step_time_1=5, Step_time_2=20, Init_val=0, New_val=1}
      mask prompts: Step_time_1 "Step time 1:"; Step_time_2 "Step time 2:"; Init_val "Inital Value:"; New_val "New Value:"
      mask Display: plot([1 2 3 4 4 5 6 7 7 8 9 10],[0 0 0 0 1 1 1 1 0 0 0 0]);
  Subsystem16 : Subsystem  mask{Step_time_1=35, Step_time_2=50, Init_val=0, New_val=1}
      mask prompts: Step_time_1 "Step time 1:"; Step_time_2 "Step time 2:"; Init_val "Inital Value:"; New_val "New Value:"
      mask Display: plot([1 2 3 4 4 5 6 7 7 8 9 10],[0 0 0 0 1 1 1 1 0 0 0 0]);
  Subsystem2 : Subsystem  mask{Step_time_1=95, Step_time_2=110, Init_val=0, New_val=pi/12}
      mask prompts: Step_time_1 "Step time 1:"; Step_time_2 "Step time 2:"; Init_val "Inital Value:"; New_val "New Value:"
      mask Display: plot([1 2 3 4 4 5 6 7 7 8 9 10],[0 0 0 0 1 1 1 1 0 0 0 0]);
  Subsystem3 : Subsystem  mask{Step_time_1=125, Step_time_2=140, Init_val=0, New_val=pi/12}
      mask prompts: Step_time_1 "Step time 1:"; Step_time_2 "Step time 2:"; Init_val "Inital Value:"; New_val "New Value:"
      mask Display: plot([1 2 3 4 4 5 6 7 7 8 9 10],[0 0 0 0 1 1 1 1 0 0 0 0]);
  Subsystem4 : Subsystem  mask{Step_time_1=155, Step_time_2=170, Init_val=0, New_val=pi/12}
      mask prompts: Step_time_1 "Step time 1:"; Step_time_2 "Step time 2:"; Init_val "Inital Value:"; New_val "New Value:"
      mask Display: plot([1 2 3 4 4 5 6 7 7 8 9 10],[0 0 0 0 1 1 1 1 0 0 0 0]);
  Subsystem6 : Subsystem  mask{Step_time_1=5, Step_time_2=20, Init_val=0, New_val=1}
      mask prompts: Step_time_1 "Step time 1:"; Step_time_2 "Step time 2:"; Init_val "Inital Value:"; New_val "New Value:"
      mask Display: plot([1 2 3 4 4 5 6 7 7 8 9 10],[0 0 0 0 1 1 1 1 0 0 0 0]);
  Subsystem8 : Subsystem  mask{Step_time_1=35, Step_time_2=50, Init_val=0, New_val=pi/12}
      mask prompts: Step_time_1 "Step time 1:"; Step_time_2 "Step time 2:"; Init_val "Inital Value:"; New_val "New Value:"
      mask Display: plot([1 2 3 4 4 5 6 7 7 8 9 10],[0 0 0 0 1 1 1 1 0 0 0 0]);
  Subsystem9 : Subsystem  mask{Step_time_1=65, Step_time_2=80, Init_val=0, New_val=pi/12}
      mask prompts: Step_time_1 "Step time 1:"; Step_time_2 "Step time 2:"; Init_val "Inital Value:"; New_val "New Value:"
      mask Display: plot([1 2 3 4 4 5 6 7 7 8 9 10],[0 0 0 0 1 1 1 1 0 0 0 0]);
  eta_ref : Outport
  wires:
  Subsystem15/1(Out1) -> Mux1/1
  Subsystem16/1(Out1) -> Mux1/2
  Subsystem1/1(Out1) -> Mux1/3
  Subsystem2/1(Out1) -> Mux2/1
  Subsystem3/1(Out1) -> Mux2/2
  Subsystem4/1(Out1) -> Mux2/3
  Mux/1 -> Manual Switch/2
  Subsystem8/1(Out1) -> Mux4/1
  Subsystem9/1(Out1) -> Mux4/2
  Constant2/1 -> Mux4/3
  Constant/1 -> Mux3/1
  Rate Limiter4/1 -> Mux5/2
  Rate Limiter1/1 -> Mux5/1
  Mux4/1 -> Rate Limiter4/1
  Mux3/1 -> Rate Limiter1/1
  Mux5/1 -> Manual Switch/1
  Constant1/1 -> Mux3/2
  Subsystem6/1(Out1) -> Mux3/3
  Rate Limiter3/1 -> Mux/2
  Mux2/1 -> Rate Limiter3/1
  Mux1/1 -> Rate Limiter2/1
  Rate Limiter2/1 -> Mux/1
  Manual Switch1/1 -> eta_ref/1
  Constant3/1 -> Manual Switch1/1
  Manual Switch/1 -> Manual Switch1/2

== system modelsimulator/Subsystem ==
  Ref : Inport
  PID : Inport  Port=2
  LQR : Inport  Port=3
  SMC : Inport  Port=4
  Demux{,1..3} (4 alike) : Demux  Outputs=6
  Mux{,1..5} (6 alike) : Mux
  Out1 : Outport
  Out2 : Outport  Port=2
  Out3 : Outport  Port=3
  Out4 : Outport  Port=4
  Out5 : Outport  Port=5
  Out6 : Outport  Port=6
  wires:
  Demux/4 -> Mux3/1  "Ref"
  Demux/5 -> Mux4/1  "Ref"
  Demux/6 -> Mux5/1  "Ref"
  Demux/1 -> Mux/1  "Ref"
  Demux/2 -> Mux1/1  "Ref"
  Ref/1 -> Demux/1
  Demux/3 -> Mux2/1  "Ref"
  Mux/1 -> Out1/1
  Mux1/1 -> Out2/1
  Mux2/1 -> Out3/1
  Mux5/1 -> Out6/1
  Mux4/1 -> Out5/1
  Mux3/1 -> Out4/1
  PID/1 -> Demux1/1
  Demux1/1 -> Mux/2  "PID"
  Demux1/2 -> Mux1/2  "PID"
  Demux1/3 -> Mux2/2  "PID"
  Demux1/4 -> Mux3/2  "PID"
  Demux1/5 -> Mux4/2  "PID"
  Demux1/6 -> Mux5/2  "PID"
  Demux2/1 -> Mux/3  "LQR"
  Demux2/2 -> Mux1/3  "LQR"
  Demux2/3 -> Mux2/3  "LQR"
  Demux2/4 -> Mux3/3  "LQR"
  Demux2/5 -> Mux4/3  "LQR"
  Demux2/6 -> Mux5/3  "LQR"
  Demux3/1 -> Mux/4  "SMC"
  Demux3/2 -> Mux1/4  "SMC"
  Demux3/3 -> Mux2/4  "SMC"
  Demux3/4 -> Mux3/4  "SMC"
  Demux3/5 -> Mux4/4  "SMC"
  Demux3/6 -> Mux5/4  "SMC"
  LQR/1 -> Demux2/1
  SMC/1 -> Demux3/1

== system modelsimulator/Subsystem1 ==
  Ref : Inport
  PID : Inport  Port=2
  LQR : Inport  Port=3
  SMC : Inport  Port=4
  Demux{,1..3} (4 alike) : Demux  Outputs=6
  Mux{,1..5} (6 alike) : Mux
  Out1 : Outport
  Out2 : Outport  Port=2
  Out3 : Outport  Port=3
  Out4 : Outport  Port=4
  Out5 : Outport  Port=5
  Out6 : Outport  Port=6
  wires:
  Demux/4 -> Mux3/1  "Ref"
  Demux/5 -> Mux4/1  "Ref"
  Demux/6 -> Mux5/1  "Ref"
  Demux/1 -> Mux/1  "Ref"
  Demux/2 -> Mux1/1  "Ref"
  Ref/1 -> Demux/1
  Demux/3 -> Mux2/1  "Ref"
  Mux/1 -> Out1/1
  Mux1/1 -> Out2/1
  Mux2/1 -> Out3/1
  Mux5/1 -> Out6/1
  Mux4/1 -> Out5/1
  Mux3/1 -> Out4/1
  PID/1 -> Demux1/1
  Demux1/1 -> Mux/2  "PID"
  Demux1/2 -> Mux1/2  "PID"
  Demux1/3 -> Mux2/2  "PID"
  Demux1/4 -> Mux3/2  "PID"
  Demux1/5 -> Mux4/2  "PID"
  Demux1/6 -> Mux5/2  "PID"
  Demux2/1 -> Mux/3  "LQR"
  Demux2/2 -> Mux1/3  "LQR"
  Demux2/3 -> Mux2/3  "LQR"
  Demux2/4 -> Mux3/3  "LQR"
  Demux2/5 -> Mux4/3  "LQR"
  Demux2/6 -> Mux5/3  "LQR"
  Demux3/1 -> Mux/4  "SMC"
  Demux3/2 -> Mux1/4  "SMC"
  Demux3/3 -> Mux2/4  "SMC"
  Demux3/4 -> Mux3/4  "SMC"
  Demux3/5 -> Mux4/4  "SMC"
  Demux3/6 -> Mux5/4  "SMC"
  LQR/1 -> Demux2/1
  SMC/1 -> Demux3/1

== system modelsimulator/Subsystem12 ==
  Ref : Inport
  PID : Inport  Port=2
  LQR : Inport  Port=3
  SMC : Inport  Port=4
  Demux{,1..3} (4 alike) : Demux  Outputs=6
  Mux{,1..5} (6 alike) : Mux
  Out1 : Outport
  Out2 : Outport  Port=2
  Out3 : Outport  Port=3
  Out4 : Outport  Port=4
  Out5 : Outport  Port=5
  Out6 : Outport  Port=6
  wires:
  SMC/1 -> Demux3/1
  LQR/1 -> Demux2/1
  Demux3/6 -> Mux5/4  "SMC"
  Demux3/5 -> Mux4/4  "SMC"
  Demux3/4 -> Mux3/4  "SMC"
  Demux3/3 -> Mux2/4  "SMC"
  Demux3/2 -> Mux1/4  "SMC"
  Demux3/1 -> Mux/4  "SMC"
  Demux2/6 -> Mux5/3  "LQR"
  Demux2/5 -> Mux4/3  "LQR"
  Demux2/4 -> Mux3/3  "LQR"
  Demux2/3 -> Mux2/3  "LQR"
  Demux2/2 -> Mux1/3  "LQR"
  Demux2/1 -> Mux/3  "LQR"
  Demux1/6 -> Mux5/2  "PID"
  Demux1/5 -> Mux4/2  "PID"
  Demux1/4 -> Mux3/2  "PID"
  Demux1/3 -> Mux2/2  "PID"
  Demux1/2 -> Mux1/2  "PID"
  Demux1/1 -> Mux/2  "PID"
  PID/1 -> Demux1/1
  Mux3/1 -> Out4/1
  Mux4/1 -> Out5/1
  Mux5/1 -> Out6/1
  Mux2/1 -> Out3/1
  Mux1/1 -> Out2/1
  Mux/1 -> Out1/1
  Demux/3 -> Mux2/1  "Ref"
  Ref/1 -> Demux/1
  Demux/2 -> Mux1/1  "Ref"
  Demux/1 -> Mux/1  "Ref"
  Demux/6 -> Mux5/1  "Ref"
  Demux/5 -> Mux4/1  "Ref"
  Demux/4 -> Mux3/1  "Ref"

== system modelsimulator/Subsystem13 ==
  Ref : Inport
  PID : Inport  Port=2
  LQR : Inport  Port=3
  SMC : Inport  Port=4
  Demux{,1..3} (4 alike) : Demux  Outputs=6
  Mux{,1..5} (6 alike) : Mux
  Out1 : Outport
  Out2 : Outport  Port=2
  Out3 : Outport  Port=3
  Out4 : Outport  Port=4
  Out5 : Outport  Port=5
  Out6 : Outport  Port=6
  wires:
  Demux/4 -> Mux3/1  "Ref"
  Demux/5 -> Mux4/1  "Ref"
  Demux/6 -> Mux5/1  "Ref"
  Demux/1 -> Mux/1  "Ref"
  Demux/2 -> Mux1/1  "Ref"
  Ref/1 -> Demux/1
  Demux/3 -> Mux2/1  "Ref"
  Mux/1 -> Out1/1
  Mux1/1 -> Out2/1
  Mux2/1 -> Out3/1
  Mux5/1 -> Out6/1
  Mux4/1 -> Out5/1
  Mux3/1 -> Out4/1
  PID/1 -> Demux1/1
  Demux1/1 -> Mux/2  "PID"
  Demux1/2 -> Mux1/2  "PID"
  Demux1/3 -> Mux2/2  "PID"
  Demux1/4 -> Mux3/2  "PID"
  Demux1/5 -> Mux4/2  "PID"
  Demux1/6 -> Mux5/2  "PID"
  Demux2/1 -> Mux/3  "LQR"
  Demux2/2 -> Mux1/3  "LQR"
  Demux2/3 -> Mux2/3  "LQR"
  Demux2/4 -> Mux3/3  "LQR"
  Demux2/5 -> Mux4/3  "LQR"
  Demux2/6 -> Mux5/3  "LQR"
  Demux3/1 -> Mux/4  "SMC"
  Demux3/2 -> Mux1/4  "SMC"
  Demux3/3 -> Mux2/4  "SMC"
  Demux3/4 -> Mux3/4  "SMC"
  Demux3/5 -> Mux4/4  "SMC"
  Demux3/6 -> Mux5/4  "SMC"
  LQR/1 -> Demux2/1
  SMC/1 -> Demux3/1

== system modelsimulator/Subsystem2 ==
  u : Inport
  Abs : Abs  SaturateOnIntegerOverflow=off
  Add : Sum  Inputs=++++++++
  Constant1 : Constant  Value=ThrusterVoltage
  Demux : Demux  Outputs=8
  Integrator : Integrator
  MATLAB Function9 : MATLAB Function  TreatAsAtomicUnit=on
  Saturation : Saturate  UpperLimit=1  LowerLimit=-1  ZeroCross=off
      settings: LockScale=on
  F_tot : Outport
  wires:
  Saturation/1 -> MATLAB Function9/1(u)
  Constant1/1 -> MATLAB Function9/2(Thruster_voltage)
  u/1 -> Saturation/1
  MATLAB Function9/1(F) -> Abs/1
  Demux/1 -> Add/1
  Demux/2 -> Add/2
  Demux/3 -> Add/3
  Demux/4 -> Add/4
  Demux/5 -> Add/5
  Demux/6 -> Add/6
  Demux/7 -> Add/7
  Demux/8 -> Add/8
  Abs/1 -> Integrator/1
  Integrator/1 -> Demux/1
  Add/1 -> F_tot/1

== system modelsimulator/Subsystem3 ==
  u : Inport
  Abs : Abs  SaturateOnIntegerOverflow=off
  Add : Sum  Inputs=++++++++
  Constant1 : Constant  Value=ThrusterVoltage
  Demux : Demux  Outputs=8
  Integrator : Integrator
  MATLAB Function9 : MATLAB Function  TreatAsAtomicUnit=on
  Saturation : Saturate  UpperLimit=1  LowerLimit=-1  ZeroCross=off
      settings: LockScale=on
  F_tot : Outport
  wires:
  Saturation/1 -> MATLAB Function9/1(u)
  Constant1/1 -> MATLAB Function9/2(Thruster_voltage)
  u/1 -> Saturation/1
  MATLAB Function9/1(F) -> Abs/1
  Demux/1 -> Add/1
  Demux/2 -> Add/2
  Demux/3 -> Add/3
  Demux/4 -> Add/4
  Demux/5 -> Add/5
  Demux/6 -> Add/6
  Demux/7 -> Add/7
  Demux/8 -> Add/8
  Abs/1 -> Integrator/1
  Integrator/1 -> Demux/1
  Add/1 -> F_tot/1

== system modelsimulator/Subsystem4 ==
  u : Inport
  Abs : Abs  SaturateOnIntegerOverflow=off
  Add : Sum  Inputs=++++++++
  Constant1 : Constant  Value=ThrusterVoltage
  Demux : Demux  Outputs=8
  Integrator : Integrator
  MATLAB Function9 : MATLAB Function  TreatAsAtomicUnit=on
  Saturation : Saturate  UpperLimit=1  LowerLimit=-1  ZeroCross=off
      settings: LockScale=on
  F_tot : Outport
  wires:
  Saturation/1 -> MATLAB Function9/1(u)
  Constant1/1 -> MATLAB Function9/2(Thruster_voltage)
  u/1 -> Saturation/1
  MATLAB Function9/1(F) -> Abs/1
  Demux/1 -> Add/1
  Demux/2 -> Add/2
  Demux/3 -> Add/3
  Demux/4 -> Add/4
  Demux/5 -> Add/5
  Demux/6 -> Add/6
  Demux/7 -> Add/7
  Demux/8 -> Add/8
  Abs/1 -> Integrator/1
  Integrator/1 -> Demux/1
  Add/1 -> F_tot/1

== system modelsimulator/Thrusters_model1 ==
  u : Inport
  Constant : Constant  Value=Enable_dynamics
  Constant1 : Constant  Value=Thruster_voltage
  Constant7 : Constant  Value=ROV.T
  MATLAB Function9 : MATLAB Function  TreatAsAtomicUnit=on
  Matrix Multiply : Product  Multiplication=Matrix(*)
  Saturation : Saturate  UpperLimit=1  LowerLimit=-1  ZeroCross=off
      settings: LockScale=on
  Subsystem : Subsystem
  Subsystem1 : Subsystem  Commented=on
  Switch : Switch  Criteria=u2 > Threshold  RndMeth=Simplest  SaturateOnIntegerOverflow=off  InputSameDT=off
  tau : Outport
  wires:
  u/1 -> Saturation/1
  Saturation/1 -> MATLAB Function9/1(u)
  Constant/1 -> Switch/2
  Constant1/1 -> MATLAB Function9/2(Thruster_voltage)
  Constant7/1 -> Matrix Multiply/1
  Switch/1 -> Matrix Multiply/2
  Matrix Multiply/1 -> tau/1
  MATLAB Function9/1(F) -> Subsystem/1(F), Switch/3
  Subsystem/1(Out1) -> Switch/1

== system modelsimulator/Thrusters_model2 ==
  u : Inport
  Constant : Constant  Value=Enable_dynamics
  Constant1 : Constant  Value=Thruster_voltage
  Constant7 : Constant  Value=ROV.T
  MATLAB Function9 : MATLAB Function  TreatAsAtomicUnit=on
  Matrix Multiply : Product  Multiplication=Matrix(*)
  Saturation : Saturate  UpperLimit=1  LowerLimit=-1  ZeroCross=off
      settings: LockScale=on
  Subsystem : Subsystem
  Subsystem1 : Subsystem  Commented=on
  Switch : Switch  Criteria=u2 > Threshold  RndMeth=Simplest  SaturateOnIntegerOverflow=off  InputSameDT=off
  tau : Outport
  wires:
  Matrix Multiply/1 -> tau/1
  Switch/1 -> Matrix Multiply/2
  Constant7/1 -> Matrix Multiply/1
  Constant1/1 -> MATLAB Function9/2(Thruster_voltage)
  Constant/1 -> Switch/2
  Saturation/1 -> MATLAB Function9/1(u)
  u/1 -> Saturation/1
  MATLAB Function9/1(F) -> Subsystem/1(F), Switch/3
  Subsystem/1(Out1) -> Switch/1

== system modelsimulator/Thrusters_model3 ==
  u : Inport
  Constant : Constant  Value=Enable_dynamics
  Constant1 : Constant  Value=Thruster_voltage
  Constant7 : Constant  Value=ROV.T
  MATLAB Function9 : MATLAB Function  TreatAsAtomicUnit=on
  Matrix Multiply : Product  Multiplication=Matrix(*)
  Saturation : Saturate  UpperLimit=1  LowerLimit=-1  ZeroCross=off
      settings: LockScale=on
  Subsystem : Subsystem
  Subsystem2 : Subsystem  Commented=on
  Switch : Switch  Criteria=u2 > Threshold  RndMeth=Simplest  SaturateOnIntegerOverflow=off  InputSameDT=off
  tau : Outport
  wires:
  Matrix Multiply/1 -> tau/1
  Switch/1 -> Matrix Multiply/2
  Constant7/1 -> Matrix Multiply/1
  Constant1/1 -> MATLAB Function9/2(Thruster_voltage)
  Constant/1 -> Switch/2
  Saturation/1 -> MATLAB Function9/1(u)
  u/1 -> Saturation/1
  MATLAB Function9/1(F) -> Subsystem/1(F), Switch/3
  Subsystem/1(Out1) -> Switch/1

== system modelsimulator/Disturbanses/Subsystem1 ==
  Step : Step  Time=Step_time_1  Before=Init_val  After=New_val  SampleTime=0
  Step1 : Step  Time=Step_time_2  After=New_val  SampleTime=0
  Sum : Sum  Inputs=|+-
  Out1 : Outport
  wires:
  Step1/1 -> Sum/2
  Step/1 -> Sum/1
  Sum/1 -> Out1/1

== system modelsimulator/Disturbanses/Subsystem10 ==
  Step : Step  Time=Step_time_1  Before=Init_val  After=New_val  SampleTime=0
  Step1 : Step  Time=Step_time_2  After=New_val  SampleTime=0
  Sum : Sum  Inputs=|+-
  Out1 : Outport
  wires:
  Sum/1 -> Out1/1
  Step/1 -> Sum/1
  Step1/1 -> Sum/2

== system modelsimulator/Disturbanses/Subsystem11 ==
  Step : Step  Time=Step_time_1  Before=Init_val  After=New_val  SampleTime=0
  Step1 : Step  Time=Step_time_2  After=New_val  SampleTime=0
  Sum : Sum  Inputs=|+-
  Out1 : Outport
  wires:
  Step1/1 -> Sum/2
  Step/1 -> Sum/1
  Sum/1 -> Out1/1

== system modelsimulator/Disturbanses/Subsystem12 ==
  Step : Step  Time=Step_time_1  Before=Init_val  After=New_val  SampleTime=0
  Step1 : Step  Time=Step_time_2  After=New_val  SampleTime=0
  Sum : Sum  Inputs=|+-
  Out1 : Outport
  wires:
  Sum/1 -> Out1/1
  Step/1 -> Sum/1
  Step1/1 -> Sum/2

== system modelsimulator/Disturbanses/Subsystem13 ==
  Step : Step  Time=Step_time_1  Before=Init_val  After=New_val  SampleTime=0
  Step1 : Step  Time=Step_time_2  After=New_val  SampleTime=0
  Sum : Sum  Inputs=|+-
  Out1 : Outport
  wires:
  Sum/1 -> Out1/1
  Step/1 -> Sum/1
  Step1/1 -> Sum/2

== system modelsimulator/Disturbanses/Subsystem14 ==
  Step : Step  Time=Step_time_1  Before=Init_val  After=New_val  SampleTime=0
  Step1 : Step  Time=Step_time_2  After=New_val  SampleTime=0
  Sum : Sum  Inputs=|+-
  Out1 : Outport
  wires:
  Step1/1 -> Sum/2
  Step/1 -> Sum/1
  Sum/1 -> Out1/1

== system modelsimulator/Disturbanses/Subsystem15 ==
  Step : Step  Time=Step_time_1  Before=Init_val  After=New_val  SampleTime=0
  Step1 : Step  Time=Step_time_2  After=New_val  SampleTime=0
  Sum : Sum  Inputs=|+-
  Out1 : Outport
  wires:
  Sum/1 -> Out1/1
  Step/1 -> Sum/1
  Step1/1 -> Sum/2

== system modelsimulator/Disturbanses/Subsystem16 ==
  Step : Step  Time=Step_time_1  Before=Init_val  After=New_val  SampleTime=0
  Step1 : Step  Time=Step_time_2  After=New_val  SampleTime=0
  Sum : Sum  Inputs=|+-
  Out1 : Outport
  wires:
  Sum/1 -> Out1/1
  Step/1 -> Sum/1
  Step1/1 -> Sum/2

== system modelsimulator/Disturbanses/Subsystem17 ==
  Step : Step  Time=Step_time_1  Before=Init_val  After=New_val  SampleTime=0
  Step1 : Step  Time=Step_time_2  After=New_val  SampleTime=0
  Sum : Sum  Inputs=|+-
  Out1 : Outport
  wires:
  Sum/1 -> Out1/1
  Step/1 -> Sum/1
  Step1/1 -> Sum/2

== system modelsimulator/Disturbanses/Subsystem2 ==
  Step : Step  Time=Step_time_1  Before=Init_val  After=New_val  SampleTime=0
  Step1 : Step  Time=Step_time_2  After=New_val  SampleTime=0
  Sum : Sum  Inputs=|+-
  Out1 : Outport
  wires:
  Sum/1 -> Out1/1
  Step/1 -> Sum/1
  Step1/1 -> Sum/2

== system modelsimulator/Disturbanses/Subsystem3 ==
  Step : Step  Time=Step_time_1  Before=Init_val  After=New_val  SampleTime=0
  Step1 : Step  Time=Step_time_2  After=New_val  SampleTime=0
  Sum : Sum  Inputs=|+-
  Out1 : Outport
  wires:
  Step1/1 -> Sum/2
  Step/1 -> Sum/1
  Sum/1 -> Out1/1

== system modelsimulator/Disturbanses/Subsystem4 ==
  Step : Step  Time=Step_time_1  Before=Init_val  After=New_val  SampleTime=0
  Step1 : Step  Time=Step_time_2  After=New_val  SampleTime=0
  Sum : Sum  Inputs=|+-
  Out1 : Outport
  wires:
  Sum/1 -> Out1/1
  Step/1 -> Sum/1
  Step1/1 -> Sum/2

== system modelsimulator/Disturbanses/Subsystem5 ==
  Step : Step  Time=Step_time_1  Before=Init_val  After=New_val  SampleTime=0
  Step1 : Step  Time=Step_time_2  After=New_val  SampleTime=0
  Sum : Sum  Inputs=|+-
  Out1 : Outport
  wires:
  Step1/1 -> Sum/2
  Step/1 -> Sum/1
  Sum/1 -> Out1/1

== system modelsimulator/Disturbanses/Subsystem6 ==
  Step : Step  Time=Step_time_1  Before=Init_val  After=New_val  SampleTime=0
  Step1 : Step  Time=Step_time_2  After=New_val  SampleTime=0
  Sum : Sum  Inputs=|+-
  Out1 : Outport
  wires:
  Sum/1 -> Out1/1
  Step/1 -> Sum/1
  Step1/1 -> Sum/2

== system modelsimulator/Disturbanses/Subsystem7 ==
  Step : Step  Time=Step_time_1  Before=Init_val  After=New_val  SampleTime=0
  Step1 : Step  Time=Step_time_2  After=New_val  SampleTime=0
  Sum : Sum  Inputs=|+-
  Out1 : Outport
  wires:
  Sum/1 -> Out1/1
  Step/1 -> Sum/1
  Step1/1 -> Sum/2

== system modelsimulator/Disturbanses/Subsystem8 ==
  Step : Step  Time=Step_time_1  Before=Init_val  After=New_val  SampleTime=0
  Step1 : Step  Time=Step_time_2  After=New_val  SampleTime=0
  Sum : Sum  Inputs=|+-
  Out1 : Outport
  wires:
  Step1/1 -> Sum/2
  Step/1 -> Sum/1
  Sum/1 -> Out1/1

== system modelsimulator/Disturbanses/Subsystem9 ==
  Step : Step  Time=Step_time_1  Before=Init_val  After=New_val  SampleTime=0
  Step1 : Step  Time=Step_time_2  After=New_val  SampleTime=0
  Sum : Sum  Inputs=|+-
  Out1 : Outport
  wires:
  Step1/1 -> Sum/2
  Step/1 -> Sum/1
  Sum/1 -> Out1/1

== system modelsimulator/LQR_full/Force allocation ==
  Tau : Inport
  1-D Lookup Table : Lookup_n-D  NumberOfTableDimensions=1  BreakpointsForDimension1=polyval(p,[-1:0.1:1])  Table=[-1:0.1:1]  InternalRulePriority=Speed  RndMeth=Simplest
  Constant7 : Constant  Value=T_inv
  Matrix Multiply : Product  Multiplication=Matrix(*)
  u : Outport
  wires:
  Constant7/1 -> Matrix Multiply/1
  Tau/1 -> Matrix Multiply/2
  Matrix Multiply/1 -> 1-D Lookup Table/1
  1-D Lookup Table/1 -> u/1
